simulink model "test"  (R2015a)
settings: Solver=ode45  StartTime=0.0  StopTime=10.0  RelTol=1e-3
values from neighbouring files (symbols this model uses):
  mu = 5    [main.m]
  x1_0 = 4    [main.m]
  x2_0 = 10    [main.m]
settings Model: Creator=Martin  LastModifiedBy=Martin

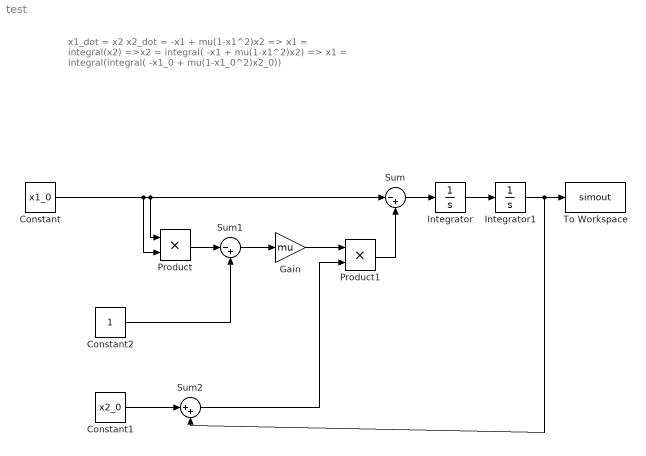
== system test ==
  note: x1_dot = x2
      | x2_dot = -x1 + mu(1-x1^2)x2
      |
      | => x1 = integral(x2)
      | =>x2 = integral( -x1 + mu(1-x1^2)x2)
      |
      | => x1 = integral(integral( -x1_0 + mu(1-x1_0^2)x2_0))
  Constant : Constant  Value=x1_0
  Constant1 : Constant  Value=x2_0
  Constant2 : Constant
  Gain : Gain  Gain=mu
  Integrator : Integrator
  Integrator1 : Integrator
  Product : Product
  Product1 : Product
  Sum : Sum  Inputs=|-+
  Sum1 : Sum  Inputs=|-+
  Sum2 : Sum  Inputs=|++
  To Workspace : ToWorkspace  VariableName=simout  SaveFormat=Timeseries  SampleTime=-1
  wires:
  Constant/1 -> Product/2, Product/1, Sum/1
  Constant2/1 -> Sum1/2
  Product/1 -> Sum1/1
  Sum1/1 -> Gain/1
  Gain/1 -> Product1/1
  Product1/1 -> Sum/2
  Sum/1 -> Integrator/1
  Integrator/1 -> Integrator1/1
  Integrator1/1 -> Sum2/2, To Workspace/1
  Sum2/1 -> Product1/2
  Constant1/1 -> Sum2/1
